simulink model "mod4"  (R2019a)
settings: Solver=VariableStepAuto  StartTime=0.0  StopTime=10.0  RelTol=1e-3
libraries: simulink x2
settings Model: Creator=step_oda  LastModifiedBy=bomjz
settings DataIOCC: ReturnWorkspaceOutputs=off
settings DebuggingCC: ArithmeticOperatorsInVariantConditions=warning
settings SFSimCC: SimUseLocalCustomCode=off
settings RTWCC: RTWUseLocalCustomCode=off
settings CodeAppCC: StateflowObjectComments=on

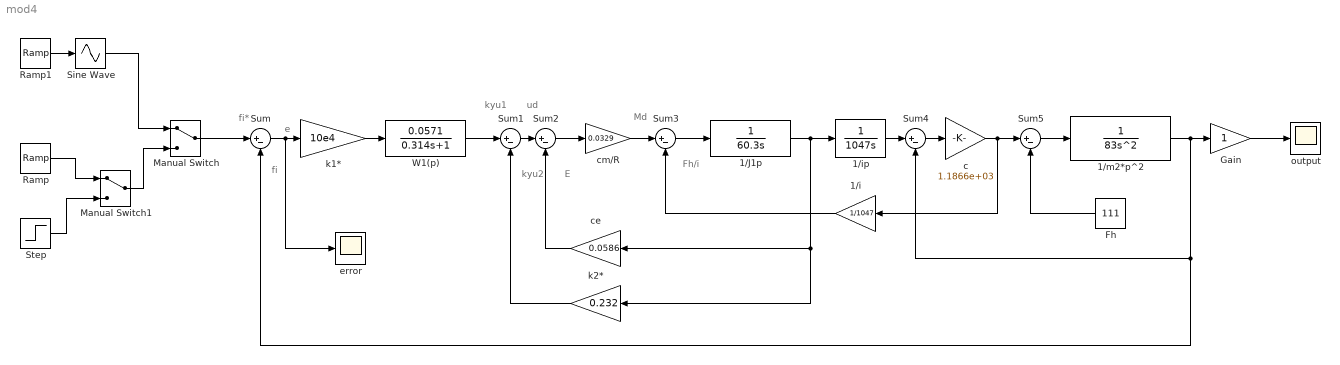
== system mod4 ==
  note: ud
  note: Md
  note: fi
  note: e
  note: fi*
  note: kyu1
  note: kyu2
  note: E
  note: Fh/i
  1/J1p : TransferFcn  Denominator=[60.3 0]
  1/i : Gain  Gain=1/1047
  1/ip : TransferFcn  Denominator=[1047 0]
  1/m2*p^2 : TransferFcn  Denominator=[83 0 0]
  Fh : Constant  Value=111
  Gain : Gain
  Manual Switch : ManualSwitch
  Manual Switch1 : ManualSwitch
  Ramp : simulink/Sources/Ramp  slope=1  start=0  InitialOutput=0
  Ramp1 : simulink/Sources/Ramp  slope=1  start=0  InitialOutput=0
  Sine Wave : Sin  TimeSource=Use external signal  Amplitude=0.09  Frequency=2  SampleTime=0
  Step : Step  Time=0  SampleTime=0
  Sum{,1..5} (6 alike) : Sum  Inputs=|+-
  W1(p) : TransferFcn  Numerator=[0.0571]  Denominator=[0.314 1]
  c : Gain  Gain=1.1866e+03
  ce : Gain  Gain=0.0586
  cm/R : Gain  Gain=0.0329
  "error " : Scope
  k1* : Gain  Gain=10e4
  k2* : Gain  Gain=0.232
  output : Scope
  wires:
  Manual Switch/1 -> Sum/1
  Sum/1 -> "error "/1, k1*/1
  k1*/1 -> W1(p)/1
  Sum1/1 -> Sum2/1
  Sum3/1 -> 1/J1p/1
  1/J1p/1 -> 1/ip/1, k2*/1, ce/1
  ce/1 -> Sum2/2
  k2*/1 -> Sum1/2
  1/i/1 -> Sum3/2
  Sum2/1 -> cm/R/1
  cm/R/1 -> Sum3/1
  Sine Wave/1 -> Manual Switch/1
  Sum5/1 -> 1/m2*p^2/1
  Sum4/1 -> c/1
  c/1 -> 1/i/1, Sum5/1
  1/ip/1 -> Sum4/1
  Fh/1 -> Sum5/2
  W1(p)/1 -> Sum1/1
  Gain/1 -> output/1
  Ramp1/1 -> Sine Wave/1
  Manual Switch1/1 -> Manual Switch/2
  Ramp/1 -> Manual Switch1/1
  Step/1 -> Manual Switch1/2
  1/m2*p^2/1 -> Sum/2, Sum4/2, Gain/1
